simulink model "DC_DC_converter"  (R2023a)
settings: Solver=VariableStepAuto  StartTime=0.0  StopTime=2  FixedStep=0.01  RelTol=1e-3
libraries: spsDiodeLib x8, spsSeriesRLCBranchLib x6, spsCurrentMeasurementLib x5, spsThyristorLib x4, spsDCVoltageSourceLib x3, spsDCMachineLib x1, spsIGBTLib x1, spsMeanLib x1, spsVoltageMeasurementLib x1, spspowerguiLib x1
settings Model: Creator=Mahdie Mohammadi  LastModifiedBy=Mahdie Mohammadi
settings SolverCC: ZeroCrossAlgorithm=Adaptive
settings DebuggingCC: IgnoredZcDiagnostic=none

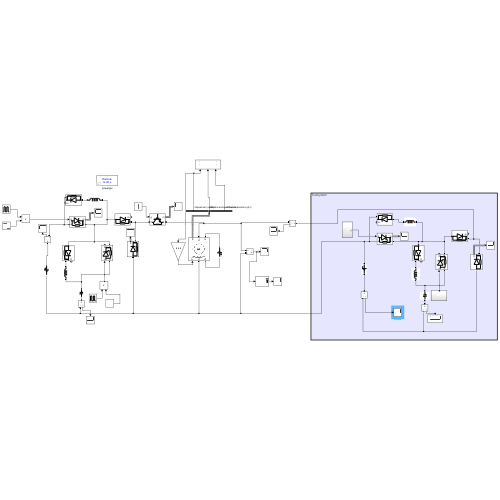
[thumbnail: Simulink's stored preview of the top-level diagram]
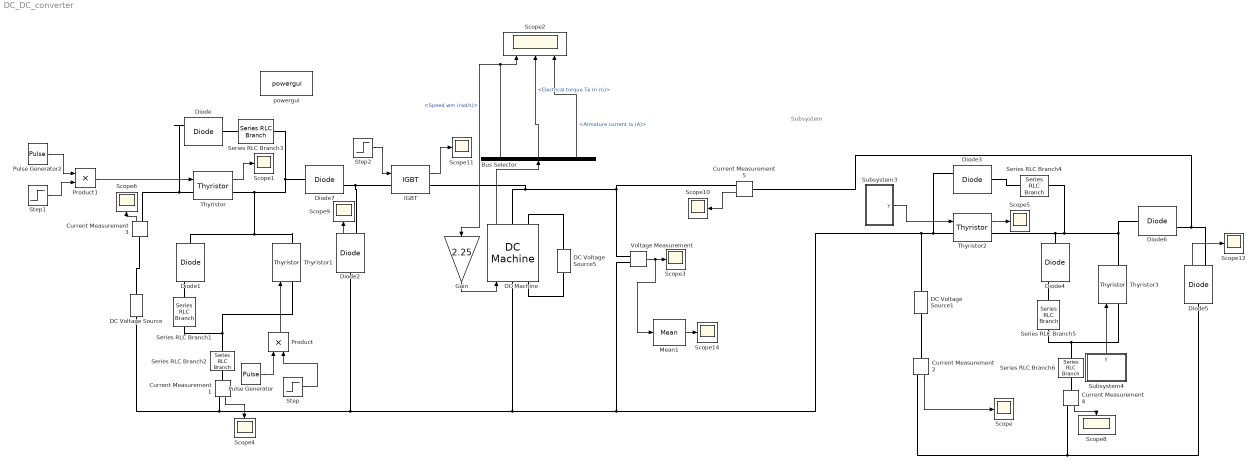
== system DC_DC_converter ==
  note: Subsystem
  Bus Selector : BusSelector  OutputSignals=Speed wm (rad/s),Electrical torque Te (n m),Armature current ia (A)
  Current Measurement{1..5} (5 alike) : spsCurrentMeasurementLib/Current Measurement  PhasorSimulation=off  OutputType=Complex  PSBequivalent=0
  DC Machine : spsDCMachineLib/DC Machine  PresetModel=07: 20HP 500V 1750RPM Field:300V  MechanicalLoad=Torque TL  FieldType=Wound  ShowDetailedParameters=on  MeasurementBus=off  RLa=[1.785 0.02124]  RLf=[105.9 27.65]  Laf=0.8413  MachineConstant=Torque constant (N.m/A)  Ke=1.8  Kt=1.8  J=0.08321  Bm=0.004313  Tf=2.105  w0=0  Ifinit=2.8328611890393  TsPowergui=0  TsBlock=-1
  DC Voltage Source : spsDCVoltageSourceLib/DC Voltage Source  Amplitude=700  Measurements=None
  DC Voltage Source1 : spsDCVoltageSourceLib/DC Voltage Source  Amplitude=700  Measurements=None
  DC Voltage Source5 : spsDCVoltageSourceLib/DC Voltage Source  Amplitude=300  Measurements=None
  Diode{,1..7} (8 alike) : spsDiodeLib/Diode  Ron=0.001  Lon=0  Vf=0.8  IC=0  UseSnubber=0  Rs=500  Cs=250e-9  Measurements=on
  Gain : Gain  Gain=2.25
  IGBT : spsIGBTLib/IGBT  Ron=0.001  Lon=0  Vf=1  Tf=1e-6  Tt=2e-6  IC=0  Rs=1e5  Cs=inf  Measurements=on
  Mean1 : spsMeanLib/Mean  Freq=60  Vinit=0  Ts=0
  Product : Product
  Product1 : Product
  Pulse Generator : DiscretePulseGenerator  PulseType=Time based  Period=1/500  PhaseDelay=(0.6)*1/500
  Pulse Generator2 : DiscretePulseGenerator  PulseType=Time based  Period=1/500  PulseWidth=2
  Scope{,1,3..6,8..12,14} (12 alike) : Scope
  Scope2 : Scope  NumInputPorts=3
  Series RLC Branch1 : spsSeriesRLCBranchLib/Series RLC Branch  LConnTagsString=__new0  RConnTagsString=__new0  BranchType=L  Resistance=1  Inductance=0.25*1e-3  SetiL0=off  InitialCurrent=0  Capacitance=1e-6  Setx0=off  InitialVoltage=0  Measurements=None
  Series RLC Branch2 : spsSeriesRLCBranchLib/Series RLC Branch  LConnTagsString=__new0  RConnTagsString=__new0  BranchType=C  Resistance=1  Inductance=1e-3  SetiL0=off  InitialCurrent=0  Capacitance=4*1e-5  Setx0=off  InitialVoltage=0  Measurements=Branch voltage
  Series RLC Branch3 : spsSeriesRLCBranchLib/Series RLC Branch  LConnTagsString=__new0  RConnTagsString=__new0  BranchType=L  Resistance=1  Inductance=0.5*1e-3  SetiL0=off  InitialCurrent=0  Capacitance=1e-6  Setx0=off  InitialVoltage=0  Measurements=None
  Series RLC Branch4 : spsSeriesRLCBranchLib/Series RLC Branch  LConnTagsString=__new0  RConnTagsString=__new0  BranchType=L  Resistance=1  Inductance=0.25*1e-3  SetiL0=off  InitialCurrent=0  Capacitance=1e-6  Setx0=off  InitialVoltage=0  Measurements=None
  Series RLC Branch5 : spsSeriesRLCBranchLib/Series RLC Branch  LConnTagsString=__new0  RConnTagsString=__new0  BranchType=L  Resistance=1  Inductance=0.25*1e-3  SetiL0=off  InitialCurrent=0  Capacitance=1e-6  Setx0=off  InitialVoltage=0  Measurements=None
  Series RLC Branch6 : spsSeriesRLCBranchLib/Series RLC Branch  LConnTagsString=__new0  RConnTagsString=__new0  BranchType=C  Resistance=1  Inductance=1e-3  SetiL0=off  InitialCurrent=0  Capacitance=1e-6  Setx0=off  InitialVoltage=0  Measurements=Branch voltage
  Step : Step  Time=0.75  Before=1  After=0  SampleTime=0
  Step1 : Step  Time=0.75  Before=1  After=0  SampleTime=0
  Step2 : Step  Time=0.75  Before=1  After=0  SampleTime=0
  Subsystem3 : Subsystem
  Subsystem4 : Subsystem
  Thyristor{,1..3} (4 alike) : spsThyristorLib/Thyristor  Ron=0.001  Lon=0  Vf=0.8  IC=0  Rs=500  Cs=250e-9  Measurements=on
  Voltage Measurement : spsVoltageMeasurementLib/Voltage Measurement  PhasorSimulation=off  OutputType=Complex  PSBequivalent=0
  powergui : spspowerguiLib/powergui  Priority=1  SimulationMode=Discrete  SampleTime=1e-6  frequency=60  Iterations=50  frequencyindice=0  Pbase=100e6  ErrMax=1e-4  UnitsV=kV  UnitsW=MW  buscounter=0  FunctionMessages=off  echomessages=off  EnableUseOfTLC=off  CurrentSourceSwitches=off  DisableSnubberDevices=off  DisableRonSwitches=off  DisableVfSwitches=off  DisplayEquations=off  AutomaticDiscreteSolvers=off  SolverType=Tustin/Backward Euler (TBE)  Interpol=off  ExternalGateDelay=off  methode=off  Ts=100  x0status=blocks  SPID=on  SwTol=0  HookPort=off  NonlinearTolerance=1e-4  nMaxIteration=100  ContinueOnMaxIteration=off  RestoreLinks=warning  ResistiveCurrentMeasurement=off  Frange=[0:2:500]  Ylog=off  Xlog=on  ShowGrid=off  save=off  variable=ZData  structure=0  ZoomFFT=off  StartTime=0.0  cycles=1  DisplayStyle=1  fundamental=60  FreqAxis=off  MaxFrequency=1000  frequencyindicesteady=1  RmsSteady=1  display=off
  wires:
  Thyristor/1 -> Scope1/1
  Current Measurement3/1 -> Scope6/1
  Gain/1 -> DC Machine/1
  Voltage Measurement/1 -> Mean1/1, Scope3/1
  Current Measurement1/1 -> Scope4/1
  DC Machine/1 -> Bus Selector/1
  Step2/1 -> IGBT/1
  IGBT/1 -> Scope11/1
  Current Measurement5/1 -> Scope10/1
  Mean1/1 -> Scope14/1
  Pulse Generator/1 -> Product/1
  Step/1 -> Product/2
  Product/1 -> Thyristor1/1
  Step1/1 -> Product1/2
  Pulse Generator2/1 -> Product1/1
  Product1/1 -> Thyristor/1
  Diode2/1 -> Scope9/1
  Thyristor2/1 -> Scope5/1
  Diode5/1 -> Scope12/1
  Current Measurement4/1 -> Scope8/1
  Subsystem3/1(y) -> Thyristor2/1
  Current Measurement2/1 -> Scope/1
  Subsystem4/1(y) -> Thyristor3/1
  Bus Selector/1 -> Scope2/1, Gain/1  "<Speed wm (rad/s)>"
  Bus Selector/2 -> Scope2/2  "<Electrical torque Te (n m)>"
  Bus Selector/3 -> Scope2/3  "<Armature current ia (A)>"
  connections:
  Series RLC Branch3/LConn1 -- Diode/LConn1
  Diode1/RConn1 -- Series RLC Branch1/LConn1
  Thyristor1/LConn1 -- Series RLC Branch2/LConn1 -- Series RLC Branch1/RConn1
  Diode/RConn1 -- Thyristor/LConn1 -- Current Measurement3/RConn1
  Series RLC Branch2/RConn1 -- Current Measurement1/LConn1
  Thyristor1/RConn1 -- Diode1/LConn1 -- Thyristor/RConn1 -- Series RLC Branch3/RConn1 -- Diode7/LConn1
  Current Measurement3/LConn1 -- DC Voltage Source/RConn1
  IGBT/RConn1 -- DC Machine/RConn1 -- Current Measurement5/RConn1 -- Voltage Measurement/LConn1
  Thyristor2/RConn1 -- Thyristor3/RConn1 -- Diode6/LConn1 -- Series RLC Branch4/LConn1 -- Diode4/LConn1
  Series RLC Branch6/LConn1 -- Thyristor3/LConn1 -- Series RLC Branch5/RConn1
  Diode5/RConn1 -- Current Measurement5/LConn1 -- Diode6/RConn1
  Current Measurement2/RConn1 -- Current Measurement4/RConn1 -- Diode5/LConn1
  Diode4/RConn1 -- Series RLC Branch5/LConn1
  Diode3/LConn1 -- Series RLC Branch4/RConn1
  Current Measurement4/LConn1 -- Series RLC Branch6/RConn1
  DC Voltage Source1/LConn1 -- Current Measurement2/LConn1
  Diode7/RConn1 -- Diode2/RConn1 -- IGBT/LConn1
  Thyristor2/LConn1 -- Diode3/RConn1 -- Voltage Measurement/LConn2 -- Diode2/LConn1 -- Current Measurement1/RConn1 -- DC Voltage Source/LConn1 -- DC Machine/LConn1 -- DC Voltage Source1/RConn1
  DC Machine/LConn2 -- DC Voltage Source5/RConn1
  DC Voltage Source5/LConn1 -- DC Machine/RConn2

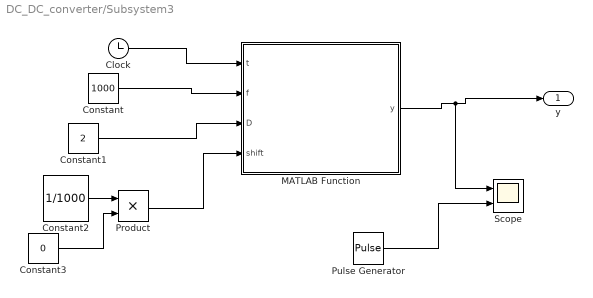
== system DC_DC_converter/Subsystem3 ==
  Clock : Clock
  Constant : Constant  Value=1000
  Constant1 : Constant  Value=2
  Constant2 : Constant  Value=1/1000
  Constant3 : Constant  Value=0
  MATLAB Function : MATLAB Function  TreatAsAtomicUnit=on
  Product : Product
  Pulse Generator : DiscretePulseGenerator  PulseType=Time based  Period=1/1000  PulseWidth=5
  Scope : Scope  NumInputPorts=2
  y : Outport
  wires:
  Clock/1 -> MATLAB Function/1(t)
  Constant2/1 -> Product/1
  Constant/1 -> MATLAB Function/2(f)
  Constant1/1 -> MATLAB Function/3(D)
  Constant3/1 -> Product/2
  Product/1 -> MATLAB Function/4(shift)
  MATLAB Function/1(y) -> Scope/1, y/1
  Pulse Generator/1 -> Scope/2

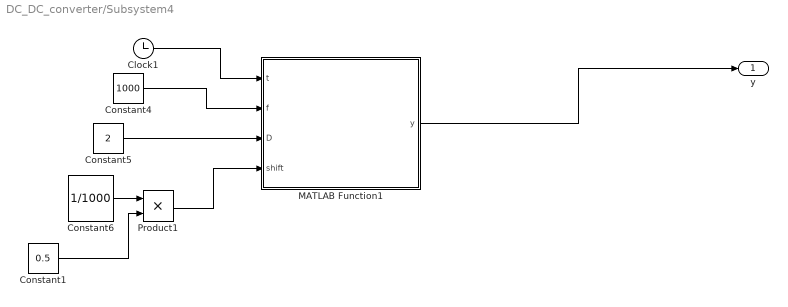
== system DC_DC_converter/Subsystem4 ==
  Clock1 : Clock
  Constant1 : Constant  Value=0.5
  Constant4 : Constant  Value=1000
  Constant5 : Constant  Value=2
  Constant6 : Constant  Value=1/1000
  MATLAB Function1 : MATLAB Function  TreatAsAtomicUnit=on
  Product1 : Product
  y : Outport
  wires:
  Constant5/1 -> MATLAB Function1/3(D)
  Constant4/1 -> MATLAB Function1/2(f)
  Constant1/1 -> Product1/2
  Constant6/1 -> Product1/1
  Product1/1 -> MATLAB Function1/4(shift)
  Clock1/1 -> MATLAB Function1/1(t)
  MATLAB Function1/1(y) -> y/1

== matlab function DC_DC_converter/Subsystem3/MATLAB Function ==
  data: t input; y output; f input; D input; shift input
function y = fcn(t,f,D,shift)
period = 1/f;
duty=D/100;
t_shift = t - shift;

 if t <= 0.75
     y = false;
 else 
     y = mod(t_shift,period) < (duty*period);

 end
end

== matlab function DC_DC_converter/Subsystem4/MATLAB Function1 ==
  data: t input; y output; f input; D input; shift input
function y = fcn(t,f,D,shift)
period = 1/f;
duty=D/100;
t_shift = t - shift;
if t < 0.75
    y = false;
   
else 
    y = mod(t_shift,period) < (duty*period);
    % y = false;
end
end
